simulink model "Ex1s"  (R2025a)
settings: Solver=VariableStepAuto  StartTime=0.0  StopTime=10.0  RelTol=1e-3
undefined symbols (not defined in the file): DiscIntNeverNeededParam, dz, nz

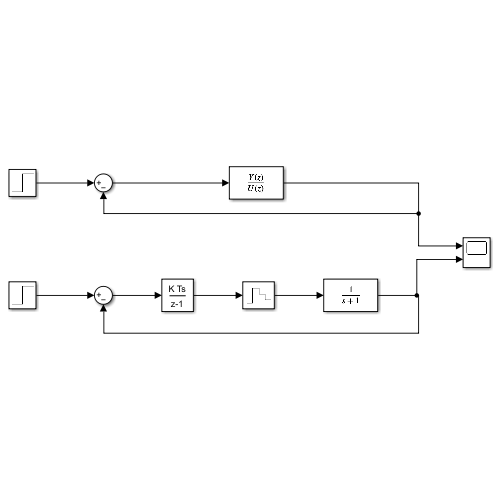
[thumbnail: Simulink's stored preview of the top-level diagram]
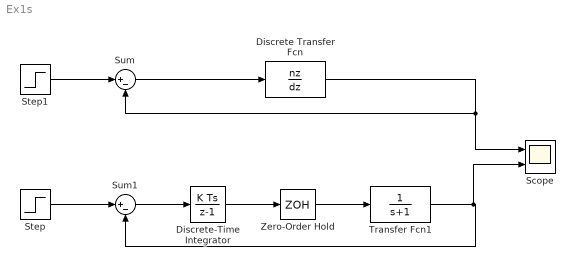
== system Ex1s ==
  Discrete Transfer Fcn : DiscreteTransferFcn  Numerator=nz  Denominator=dz
  Discrete-Time Integrator : DiscreteIntegrator  SampleTime=-1  ICPrevOutput=DiscIntNeverNeededParam  ICPrevScaledInput=DiscIntNeverNeededParam
  Scope : Scope  NumInputPorts=2
      settings: ActiveDisplayYMinimum=-0.1508431002466161  ActiveDisplayYMaximum=1.3575879022195452
  Step : Step  SampleTime=0
  Step1 : Step  SampleTime=0.1
  Sum : Sum  Inputs=|+-
  Sum1 : Sum  Inputs=|+-  SampleTime=0.1
  Transfer Fcn1 : TransferFcn  Denominator=[1 1]
  Zero-Order Hold : ZeroOrderHold  SampleTime=-1
  wires:
  Sum/1 -> Discrete Transfer Fcn/1
  Step/1 -> Sum1/1
  Sum1/1 -> Discrete-Time Integrator/1
  Discrete-Time Integrator/1 -> Zero-Order Hold/1
  Zero-Order Hold/1 -> Transfer Fcn1/1
  Transfer Fcn1/1 -> Scope/2, Sum1/2
  Discrete Transfer Fcn/1 -> Sum/2, Scope/1
  Step1/1 -> Sum/1
